simulink model "sixdofTrim"  (R2019a)
settings: Solver=VariableStepAuto  StartTime=0.0  StopTime=10.0  RelTol=1e-3
InitFcn:
  | HeightAboveSeaLevel = 5.4419142084;
  | Temperature = 288.15;
  | Pressure = 	101325;
values from neighbouring files (symbols this model uses):
  cg = temp(4)    [NonlinearStateEstimationForActuatorDelay.m]
  I = reshape(x(1:9), [3 3])    [AdaptiveLQR.m]    (also in MEKF.m = diag([0.08 0.08 0.002]); MEKFAttitudeOnly.m = diag([0.08 0.08 0.002]); MEKF_old.m = diag([0.08 0.08 0.002]); NonlinearStateEstimationForActuatorDelay.m = diag([Ixx, Ixx, Izz]))
  mass = 1.0565    [ImpactVelocityNotParallelMatlab.m]    (also in NonlinearStateEstimationForActuatorDelay.m = temp(1); OneDLanding.m; RunImpactVelocityParforCompiled.m; Tracker.m = 1.0616753546)
libraries: aerolibutil x4, simulink x4, aerolibasang x2, shared6dof x1, aerolibatmos2 x1, aerolibbdyn x1, sharedtransform x1
settings Model: Creator=rag  LastModifiedBy=rag
settings DataIOCC: ExternalInput=getinputstruct(op_trim9)  InitialState=getstatestruct(op_trim9)

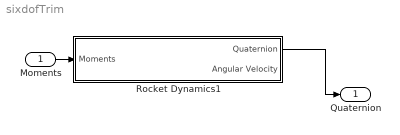
== system sixdofTrim ==
  Moments : Inport  PortDimensions=2
  Rocket Dynamics1 : Subsystem
  Quaternion : Outport
  wires:
  Rocket Dynamics1/1(Quaternion) -> Quaternion/1
  Moments/1 -> Rocket Dynamics1/1(Moments)

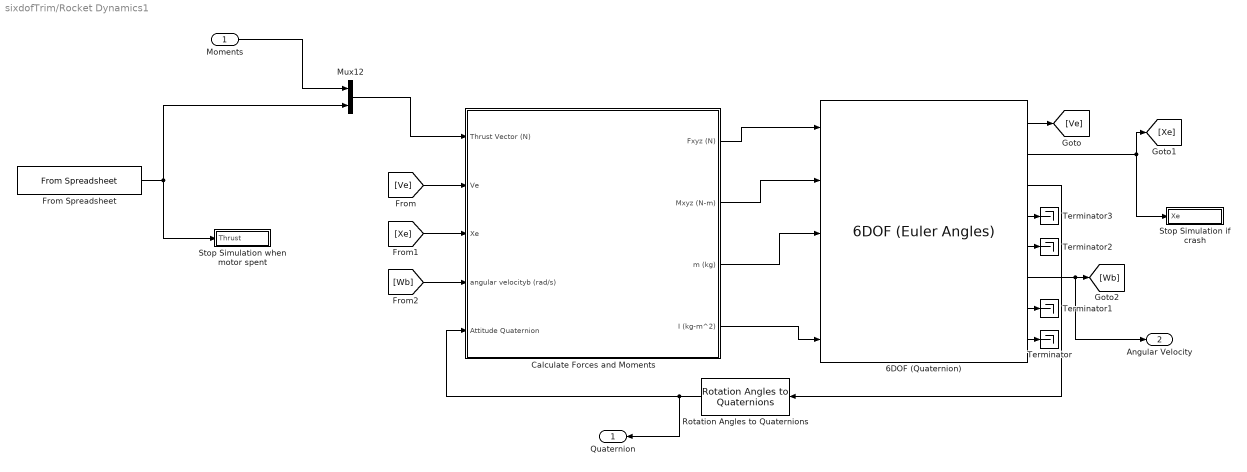
== system sixdofTrim/Rocket Dynamics1 ==
  Moments : Inport  PortDimensions=2
  6DOF (Quaternion) : shared6dof/6DOF (Euler Angles)  units=Metric (MKS)  mtype=Custom Variable  rep=Quaternion  xme_0=[0 0 0]  Vm_0=[0 0 0]  eul_0=[0 0 0]  pm_0=[0 0 0]  mass_0=1.0  mass_e=0.5  mass_f=2.0  inertia=eye(3)  inertia_e=eye(3)  inertia_f=2*eye(3)  k_quat=1.0  vre_flag=off  abi_flag=off  aMode=0  xme_statename=''  Vm_statename=''  eul_statename=''  quat_statename=''  pm_statename=''  mass_statename=''
      settings: SourceProductBaseCode=AE
  Calculate Forces and Moments : Subsystem
  From Spreadsheet : FromSpreadsheet  FileName=F10_Thrust.xls  ExtrapolationBeforeFirstDataPoint=Hold first value  ExtrapolationAfterLastDataPoint=Hold last value
  Mux12 : Mux  Inputs=2
  Rotation Angles to Quaternions : sharedtransform/Rotation Angles to Quaternions  rotationOrder=ZYX  aMode=aMode
      settings: SourceProductName=Aerospace Blockset  SourceProductBaseCode=AE
  Stop Simulation if crash : Subsystem
  Stop Simulation when motor spent : Subsystem
  Terminator{,1..3} (4 alike) : Terminator
  Quaternion : Outport
  Angular Velocity : Outport  Port=2
  wires:
  6DOF (Quaternion)/6 -> Angular Velocity/1, [Wb]
  6DOF (Quaternion)/3 -> Rotation Angles to Quaternions/1
  [Wb] -> Calculate Forces and Moments/4(angular velocityb (rad/s))
  Calculate Forces and Moments/3(m (kg)) -> 6DOF (Quaternion)/3
  6DOF (Quaternion)/2 -> Stop Simulation if crash/1(Xe), [Xe]
  6DOF (Quaternion)/4 -> Terminator3/1
  [Ve] -> Calculate Forces and Moments/2(Ve)
  6DOF (Quaternion)/7 -> Terminator1/1
  6DOF (Quaternion)/5 -> Terminator2/1
  Calculate Forces and Moments/1(Fxyz (N)) -> 6DOF (Quaternion)/1
  Calculate Forces and Moments/4(I (kg-m^2)) -> 6DOF (Quaternion)/5
  [Xe] -> Calculate Forces and Moments/3(Xe)
  Rotation Angles to Quaternions/1 -> Quaternion/1, Calculate Forces and Moments/5(Attitude Quaternion)
  6DOF (Quaternion)/1 -> [Ve]
  Calculate Forces and Moments/2(Mxyz (N-m)) -> 6DOF (Quaternion)/2
  6DOF (Quaternion)/8 -> Terminator/1
  Moments/1 -> Mux12/1
  Mux12/1 -> Calculate Forces and Moments/1(Thrust Vector (N))
  From Spreadsheet/1 -> Mux12/2, Stop Simulation when motor spent/1(Thrust)

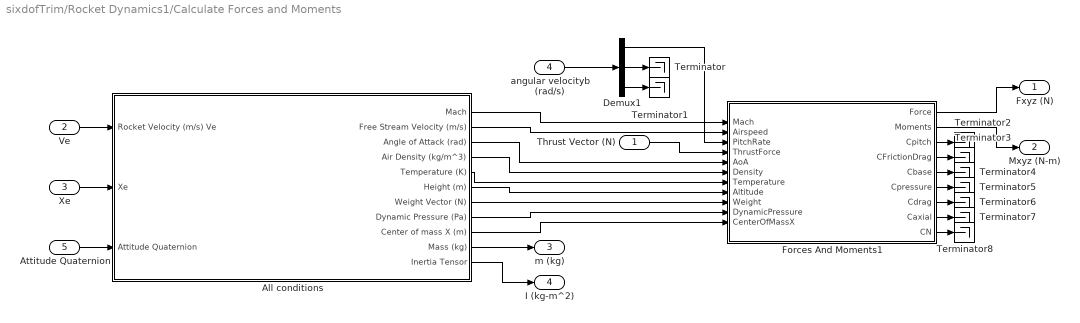
== system sixdofTrim/Rocket Dynamics1/Calculate Forces and Moments ==
  Thrust Vector (N) : Inport
  Ve : Inport  Port=2
  Xe : Inport  Port=3
  angular velocityb (rad/s) : Inport  Port=4
  Attitude Quaternion : Inport  Port=5
  All conditions : Subsystem
  Demux1 : Demux  Outputs=3
  Forces And Moments1 : MATLAB Function  TreatAsAtomicUnit=on
  Terminator{,1..8} (9 alike) : Terminator
  Fxyz (N) : Outport
  Mxyz (N-m) : Outport  Port=2
  m (kg) : Outport  Port=3
  I (kg-m^2) : Outport  Port=4
  wires:
  Demux1/1 -> Forces And Moments1/3(PitchRate)
  All conditions/11(Inertia Tensor) -> I (kg-m^2)/1
  Forces And Moments1/6(Cpressure) -> Terminator5/1
  All conditions/2(Free Stream Velocity (m/s)) -> Forces And Moments1/2(Airspeed)
  All conditions/9(Center of mass X (m)) -> Forces And Moments1/11(CenterOfMassX)
  All conditions/5(Temperature (K)) -> Forces And Moments1/7(Temperature)
  Xe/1 -> All conditions/2(Xe)
  angular velocityb (rad/s)/1 -> Demux1/1
  All conditions/3(Angle of Attack (rad)) -> Forces And Moments1/5(AoA)
  All conditions/1(Mach) -> Forces And Moments1/1(Mach)
  All conditions/4(Air Density (kg/m^3)) -> Forces And Moments1/6(Density)
  All conditions/8(Dynamic Pressure (Pa)) -> Forces And Moments1/10(DynamicPressure)
  All conditions/6(Height (m)) -> Forces And Moments1/8(Altitude)
  All conditions/7(Weight Vector (N)) -> Forces And Moments1/9(Weight)
  Forces And Moments1/1(Force) -> Fxyz (N)/1
  Forces And Moments1/2(Moments) -> Mxyz (N-m)/1
  Thrust Vector (N)/1 -> Forces And Moments1/4(ThrustForce)
  Attitude Quaternion/1 -> All conditions/3(Attitude Quaternion)
  Forces And Moments1/3(Cpitch) -> Terminator2/1
  Forces And Moments1/5(Cbase) -> Terminator4/1
  Forces And Moments1/7(Cdrag) -> Terminator6/1
  Forces And Moments1/4(CFrictionDrag) -> Terminator3/1
  Forces And Moments1/8(Caxial) -> Terminator7/1
  Ve/1 -> All conditions/1(Rocket Velocity (m/s) Ve)
  Forces And Moments1/9(CN) -> Terminator8/1
  All conditions/10(Mass (kg)) -> m (kg)/1
  Demux1/2 -> Terminator/1
  Demux1/3 -> Terminator1/1

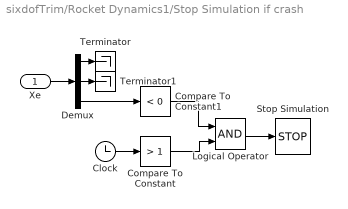
== system sixdofTrim/Rocket Dynamics1/Stop Simulation if crash ==
  Xe : Inport
  Clock : Clock
  Compare To Constant : simulink/Logic and Bit Operations/Compare To Constant  relop=>  const=1  OutDataTypeStr=boolean
  Compare To Constant1 : simulink/Logic and Bit Operations/Compare To Constant  relop=<  const=0  OutDataTypeStr=boolean
  Demux : Demux  Outputs=3
  Logical Operator : Logic  AllPortsSameDT=off  OutDataTypeStr=boolean
  Stop Simulation : Stop
  Terminator : Terminator
  Terminator1 : Terminator
  wires:
  Logical Operator/1 -> Stop Simulation/1
  Compare To Constant/1 -> Logical Operator/2
  Clock/1 -> Compare To Constant/1
  Compare To Constant1/1 -> Logical Operator/1
  Xe/1 -> Demux/1
  Demux/1 -> Terminator/1
  Demux/2 -> Terminator1/1
  Demux/3 -> Compare To Constant1/1

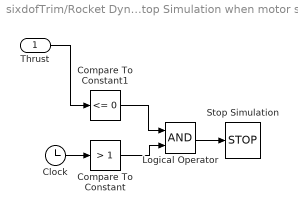
== system sixdofTrim/Rocket Dynamics1/Stop Simulation when motor spent ==
  Thrust : Inport
  Clock : Clock
  Compare To Constant : simulink/Logic and Bit Operations/Compare To Constant  relop=>  const=1  OutDataTypeStr=boolean
  Compare To Constant1 : simulink/Logic and Bit Operations/Compare To Constant  relop=<=  const=0  OutDataTypeStr=boolean
  Logical Operator : Logic  AllPortsSameDT=off  OutDataTypeStr=boolean
  Stop Simulation : Stop
  wires:
  Logical Operator/1 -> Stop Simulation/1
  Compare To Constant/1 -> Logical Operator/2
  Clock/1 -> Compare To Constant/1
  Compare To Constant1/1 -> Logical Operator/1
  Thrust/1 -> Compare To Constant1/1

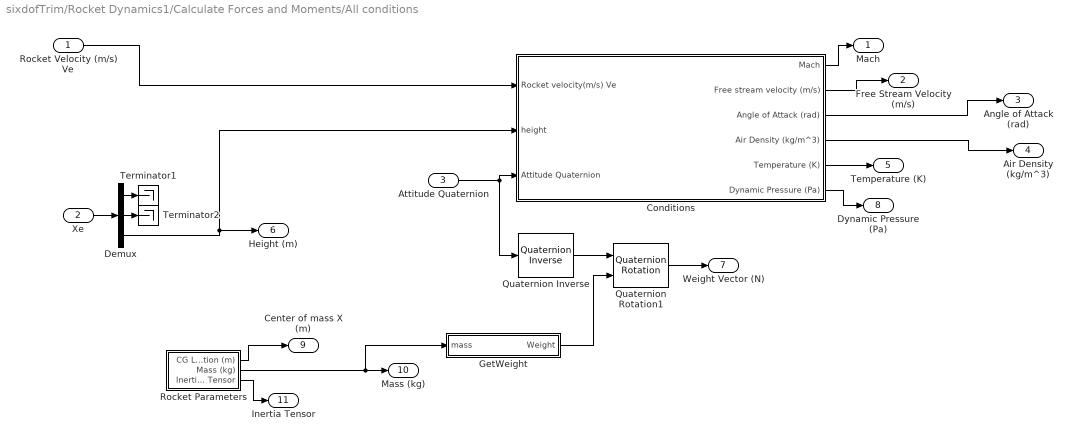
== system sixdofTrim/Rocket Dynamics1/Calculate Forces and Moments/All conditions ==
  Rocket Velocity (m/s) Ve : Inport
  Xe : Inport  Port=2
  Attitude Quaternion : Inport  Port=3
  Conditions : Subsystem
  Demux : Demux  Outputs=3
  GetWeight : MATLAB Function  TreatAsAtomicUnit=on
  Quaternion Inverse : aerolibutil/Quaternion Inverse
      settings: SourceProductName=Aerospace Blockset
  Quaternion Rotation1 : aerolibutil/Quaternion Rotation
  Rocket Parameters : Subsystem
  Terminator1 : Terminator
  Terminator2 : Terminator
  Mach : Outport
  Free Stream Velocity (m/s) : Outport  Port=2
  Angle of Attack (rad) : Outport  Port=3
  Air Density (kg/m^3) : Outport  Port=4
  Temperature (K) : Outport  Port=5
  Height (m) : Outport  Port=6
  Weight Vector (N) : Outport  Port=7
  Dynamic Pressure (Pa) : Outport  Port=8
  Center of mass X (m) : Outport  Port=9
  Mass (kg) : Outport  Port=10
  Inertia Tensor : Outport  Port=11
  wires:
  Demux/3 -> Conditions/2(height), Height (m)/1
  Conditions/4(Air Density (kg/m^3)) -> Air Density (kg/m^3)/1
  Rocket Velocity (m/s) Ve/1 -> Conditions/1(Rocket velocity(m/s) Ve)
  Conditions/5(Temperature (K)) -> Temperature (K)/1
  Conditions/1(Mach) -> Mach/1
  Conditions/2(Free stream velocity (m/s)) -> Free Stream Velocity (m/s)/1
  Demux/2 -> Terminator2/1
  GetWeight/1(Weight) -> Quaternion Rotation1/2
  Xe/1 -> Demux/1
  Rocket Parameters/1(CG Location (m)) -> Center of mass X (m)/1
  Rocket Parameters/3(Inertia Tensor) -> Inertia Tensor/1
  Quaternion Rotation1/1 -> Weight Vector (N)/1
  Conditions/3(Angle of Attack (rad)) -> Angle of Attack (rad)/1
  Demux/1 -> Terminator1/1
  Conditions/6(Dynamic Pressure (Pa)) -> Dynamic Pressure (Pa)/1
  Rocket Parameters/2(Mass (kg)) -> GetWeight/1(mass), Mass (kg)/1
  Quaternion Inverse/1 -> Quaternion Rotation1/1
  Attitude Quaternion/1 -> Quaternion Inverse/1, Conditions/3(Attitude Quaternion)

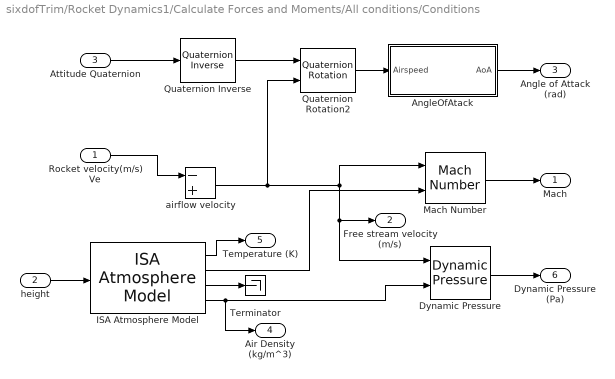
== system sixdofTrim/Rocket Dynamics1/Calculate Forces and Moments/All conditions/Conditions ==
  Rocket velocity(m/s) Ve : Inport
  height : Inport  Port=2
  Attitude Quaternion : Inport  Port=3
  AngleOfAtack : MATLAB Function  TreatAsAtomicUnit=on
  Dynamic Pressure : aerolibasang/Dynamic Pressure
  ISA Atmosphere Model : aerolibatmos2/ISA Atmosphere Model  custom=on  g=9.80665  gamma=1.4  R=287.0531  L=0.0065  h_trop=11000  h_strat=20000  rho0=1.225  P0=Pressure  T0=Temperature  h0=0
      settings: SourceProductName=Aerospace Blockset
  Mach Number : aerolibasang/Mach Number
      settings: SourceProductName=Aerospace Blockset  SourceProductBaseCode=AE
  Quaternion Inverse : aerolibutil/Quaternion Inverse
      settings: SourceProductName=Aerospace Blockset
  Quaternion Rotation2 : aerolibutil/Quaternion Rotation
  Terminator : Terminator
  airflow velocity : Sum  Inputs=-+
  Mach : Outport
  Free stream velocity (m/s) : Outport  Port=2
  Angle of Attack (rad) : Outport  Port=3
  Air Density (kg/m^3) : Outport  Port=4
  Temperature (K) : Outport  Port=5
  Dynamic Pressure (Pa) : Outport  Port=6
  wires:
  airflow velocity/1 -> Quaternion Rotation2/2, Free stream velocity (m/s)/1, Dynamic Pressure/1, Mach Number/1
  Quaternion Rotation2/1 -> AngleOfAtack/1(Airspeed)
  ISA Atmosphere Model/4 -> Dynamic Pressure/2, Air Density (kg/m^3)/1
  ISA Atmosphere Model/2 -> Mach Number/2
  Dynamic Pressure/1 -> Dynamic Pressure (Pa)/1
  ISA Atmosphere Model/3 -> Terminator/1
  Mach Number/1 -> Mach/1
  Rocket velocity(m/s) Ve/1 -> airflow velocity/1
  ISA Atmosphere Model/1 -> Temperature (K)/1
  AngleOfAtack/1(AoA) -> Angle of Attack (rad)/1
  height/1 -> ISA Atmosphere Model/1
  Attitude Quaternion/1 -> Quaternion Inverse/1
  Quaternion Inverse/1 -> Quaternion Rotation2/1

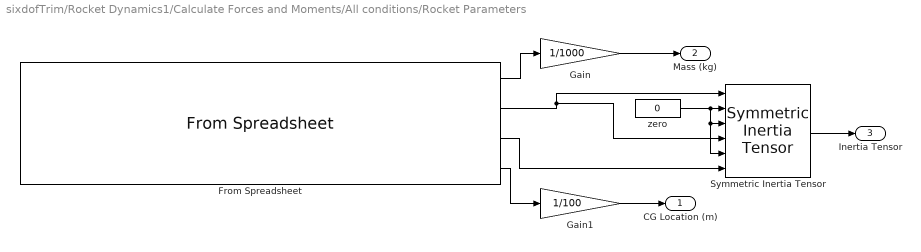
== system sixdofTrim/Rocket Dynamics1/Calculate Forces and Moments/All conditions/Rocket Parameters ==
  From Spreadsheet : FromSpreadsheet  FileName=mass,cg,I.xlsx  SheetName=mass,cg,I  Range=A1:E251  ExtrapolationBeforeFirstDataPoint=Hold first value  ExtrapolationAfterLastDataPoint=Hold last value
  Gain : Gain  Gain=1/1000
  Gain1 : Gain  Gain=1/100
  Symmetric Inertia Tensor : aerolibbdyn/Symmetric Inertia Tensor
      settings: SourceProductName=Aerospace Blockset  SourceProductBaseCode=AE
  zero : Constant  Value=0
  CG Location (m) : Outport
  Mass (kg) : Outport  Port=2
  Inertia Tensor : Outport  Port=3
  wires:
  zero/1 -> Symmetric Inertia Tensor/5, Symmetric Inertia Tensor/3, Symmetric Inertia Tensor/2
  From Spreadsheet/2 -> Symmetric Inertia Tensor/1, Symmetric Inertia Tensor/4
  From Spreadsheet/3 -> Symmetric Inertia Tensor/6
  Symmetric Inertia Tensor/1 -> Inertia Tensor/1
  From Spreadsheet/4 -> Gain1/1
  From Spreadsheet/1 -> Gain/1
  Gain/1 -> Mass (kg)/1
  Gain1/1 -> CG Location (m)/1

== matlab function sixdofTrim/Rocket Dynamics1/Calculate Forces and Moments/Forces And Moments1 ==
  settings: updateMethod=DISCRETE
  data: Mach input; Airspeed input; PitchRate input; ThrustForce input; AoA input; Density input; Temperature input; Altitude input; Weight input; Force output; DynamicPressure input; Moments output; Cpitch output; CFrictionDrag output; Cbase output; Cpressure output; Cdrag output; Caxial output; CN output; CenterOfMassX input
function [Force, Moments, Cpitch, CFrictionDrag, Cbase, Cpressure, Cdrag, Caxial, CN] = forces(Mach, Airspeed, PitchRate, ThrustForce, AoA, Density, Temperature, Altitude, Weight, DynamicPressure, CenterOfMassX)
    %% Rocket Shape Constants
    Reference_Diameter = 7.62e-2;
    Reference_Radius = Reference_Diameter / 2;
    Reference_Area = Reference_Radius^2 * pi;
    
    NoseCone_Length = 15e-2;
    BodyTube_Length = 80e-2;
    NoseCone_WetArea = pi * Reference_Radius * NoseCone_Length;          % pi*r*l
    BodyTube_WetArea = pi * Reference_Radius * 2 * BodyTube_Length;      % pi*d*l
    NoseCone_PlanformArea = Reference_Diameter * NoseCone_Length / 2;
    BodyTube_PlanformArea = Reference_Diameter * BodyTube_Length;
    
    SurfaceRoughness = 20e-6;
    
    sinphi = Reference_Radius / hypot(Reference_Radius, NoseCone_Length);
    BodyTube_CP = 0.55;
    NoseCone_CP = 0.1;
    PitchCenterX = 0;
    
    COT_to_COM = .95 - CenterOfMassX; %get actual value and change over time as solid motor burns
    
    %% General Constants
    K = 1.1;
   
    %% Coefficients
    [CN, Cpitch] = CalculatePitchAndNormalCDs(K, Reference_Diameter, AoA, Airspeed, PitchRate, NoseCone_Length, BodyTube_Length, Reference_Area, CenterOfMassX, PitchCenterX, NoseCone_PlanformArea, BodyTube_PlanformArea, NoseCone_CP, BodyTube_CP);
    
    Cbase = .12 + .13*Mach^2;
    CFrictionDrag = CalculateFrictionDrag(Temperature, Density, Reference_Radius, Reference_Area, SurfaceRoughness, NoseCone_Length, BodyTube_Length, Airspeed, Mach, NoseCone_WetArea, BodyTube_WetArea);
    Cpressure = PressureDragForce(sinphi);
    
    Cdrag = Cbase + CFrictionDrag + Cpressure;
    Caxial = AxialDragMul(AoA) * Cdrag;
    
    Cyaw = 0.0;
    
    Croll = 0;
    Cside = 0;
    
    %% Forces and Moments
    z = DynamicPressure * Reference_Area;

    Force = -z * [CN; Cside; Caxial] + ThrustForce + Weight;
    if Altitude <= 0 && Force(3) < 0
        Force(3) = 0;
    end
    
    %Thrust_moment = COT_to_COM * [ThrustForce(1); ThrustForce(2); 0];
    Thrust_moment = [ThrustForce(1); ThrustForce(2); 0];
    Moments = z * Reference_Diameter * [-Cyaw; 0.01; Croll] + Thrust_moment;
end

== matlab function sixdofTrim/Rocket Dynamics1/Calculate Forces and Moments/All conditions/Conditions/AngleOfAtack ==
  settings: updateMethod=DISCRETE
  data: Airspeed input; AoA output
function AoA = AngleOfAttack(Airspeed)
    x = -Airspeed(3) / norm(Airspeed);
    
    AoA = real(acos(complex(x))); %in case x is greater or less than one
    
    if norm(Airspeed) <= .01
        AoA = 0;
    end
end

== matlab function sixdofTrim/Rocket Dynamics1/Calculate Forces and Moments/All conditions/GetWeight ==
  settings: updateMethod=DISCRETE
  data: Weight output; mass input
function Weight  = MassToWeight(mass)
   Weight = [0; 0; -9.8065*mass];
   end
